simulink model "nonlinear_mfun"  (R2024b)
settings: Solver=ode4  StartTime=0.0  StopTime=20  FixedStep=0.01  RelTol=1e-3  AbsTol=1e-6
undefined symbols (not defined in the file): params, sim_step_gain
settings Model: Creator=david  LastModifiedBy=david

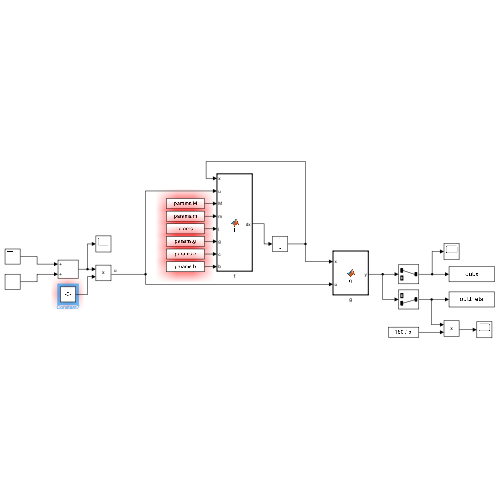
[thumbnail: Simulink's stored preview of the top-level diagram]
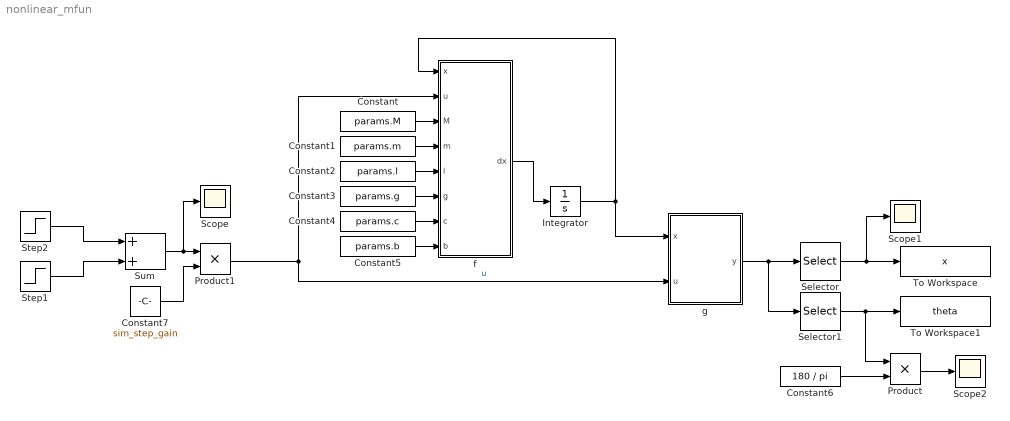
== system nonlinear_mfun ==
  Constant : Constant  Value=params.M
  Constant1 : Constant  Value=params.m
  Constant2 : Constant  Value=params.l
  Constant3 : Constant  Value=params.g
  Constant4 : Constant  Value=params.c
  Constant5 : Constant  Value=params.b
  Constant6 : Constant  Value=180 / pi
  Constant7 : Constant  Value=sim_step_gain
  Integrator : Integrator  InitialCondition=[0; 0; pi; 0]
  Product : Product
  Product1 : Product
  Scope : Scope
  Scope1 : Scope
  Scope2 : Scope
  Selector : Selector  InputPortWidth=2  IndexOptions=Index vector (dialog)  Indices=1  OutputSizes=1
  Selector1 : Selector  InputPortWidth=2  IndexOptions=Index vector (dialog)  Indices=2  OutputSizes=1
  Step1 : Step  SampleTime=0
  Step2 : Step  Time=2  After=-1  SampleTime=0
  Sum : Sum
  To Workspace : ToWorkspace  VariableName=x  SampleTime=-1
      settings: Save2DSignal=2-D array (concatenate along first dimension)
  To Workspace1 : ToWorkspace  VariableName=theta  SampleTime=-1
      settings: Save2DSignal=2-D array (concatenate along first dimension)
  f : MATLAB Function  TreatAsAtomicUnit=on
  g : MATLAB Function  TreatAsAtomicUnit=on
  wires:
  Step1/1 -> Sum/2
  Step2/1 -> Sum/1
  Sum/1 -> Product1/1, Scope/1
  Product1/1 -> f/2(u), g/2(u)  "u"
  Constant/1 -> f/3(M)
  f/1(dx) -> Integrator/1
  Integrator/1 -> g/1(x), f/1(x)
  g/1(y) -> Selector1/1, Selector/1
  Selector/1 -> To Workspace/1, Scope1/1
  Constant1/1 -> f/4(m)
  Constant2/1 -> f/5(l)
  Constant3/1 -> f/6(g)
  Constant4/1 -> f/7(c)
  Constant5/1 -> f/8(b)
  Product/1 -> Scope2/1
  Selector1/1 -> To Workspace1/1, Product/1
  Constant6/1 -> Product/2
  Constant7/1 -> Product1/2

== matlab function nonlinear_mfun/g ==
  data: x input; u input; y output
function y = g(x, u)
    y = [
        x(1); % x
        x(3); % theta
    ];
end

== matlab function nonlinear_mfun/f ==
  data: x input; u input; dx output; M input; m input; l input; g input; c input; b input
function dx = f(x, u, M, m, l, g, c, b)
    dx = [
        x(2); % dx
        (b / l * x(4) * cos(x(3)) + m * l * x(4) ^ 2 * sin(x(3)) - c * x(2) - m * g * sin(x(3)) * cos(x(3)) + u) / ...
            (M + m * sin(x(3)) ^ 2); % d2x
        x(4); % dtheta
        ((M + m) * g / l * sin(x(3)) - (M / m + 1) * b / l ^ 2 * x(4) - m * l * x(4) ^ 2 * cos(x(3)) * sin(x(3)) + c / l * x(2) * cos(x(3)) - u * cos(x(3)) / l) / ...
            (M + m * sin(x(3)) ^ 2); % d2theta
    ];
end
